simulink model "CalculateMaximumFluxLimit"  (R2026a)
settings: Solver=FixedStepDiscrete
model workspace (MAT data in the model file):
  Polepairs = Simulink.Parameter
  Polepairs.Value = 4
  Polepairs.Complexity = 'real'
  Polepairs.Dimensions = [1 1]
  Polepairs.DataType = 'auto'
settings Model: DataDictionary=TractionEmotorSoftwareArchInterfaceData.sldd  Creator=dakaihu  LastModifiedBy=dakaihu
settings OptimizationCC: GainParamInheritBuiltInType=on  UseFloatMulNetSlope=on  InlineInvariantSignals=on  NoFixptDivByZeroProtection=on  EfficientFloat2IntCast=on  LifeSpan=1
settings HardwareCC: ProdBitPerChar=16.0  ProdBitPerInt=16.0  ProdLargestAtomicInteger=Integer  ProdWordSize=16.0  ProdHWDeviceType=Texas Instruments->C2000
settings RTWCC: SystemTargetFile=ert.tlc  Description=Embedded Coder
settings CodeAppCC: MaxIdLength=60.0  CustomSymbolStrGlobalVar=rt$N$M  CustomSymbolStrType=$N$M  CustomSymbolStrFcn=$N$M$F  CustomSymbolStrMacro=$N$M
settings ERTTargetCC: ERTFilePackagingFormat=CompactWithDataFile  GenerateSampleERTMain=on  IncludeMdlTerminateFcn=off  CombineSignalStateStructs=on  SuppressErrorStatus=on  SupportAbsoluteTime=off  SupportComplex=off

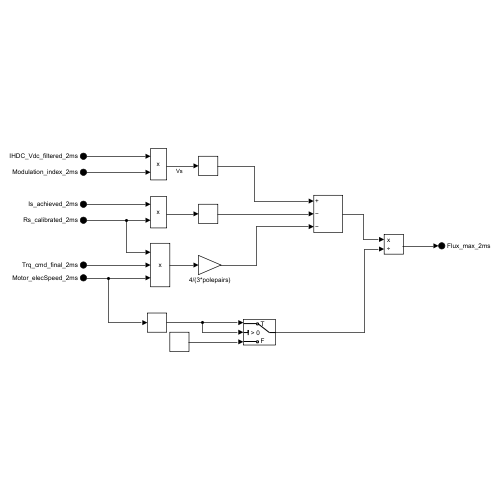
[thumbnail: Simulink's stored preview of the top-level diagram]
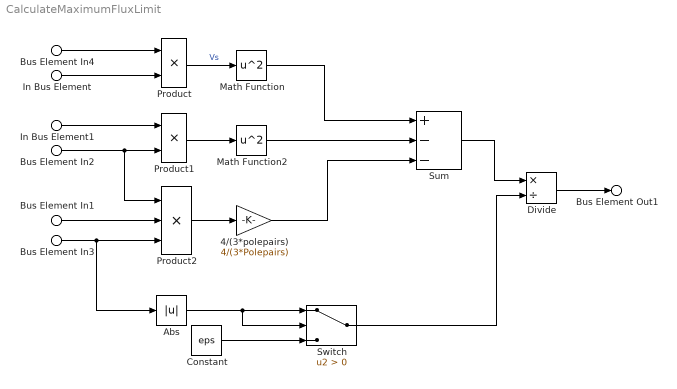
== system CalculateMaximumFluxLimit ==
  Bus Element In2 : Inport  PortName=Rs_calibrated_2ms
  Bus Element In1 : Inport  Port=2  PortName=Trq_cmd_final_2ms
  Bus Element In3 : Inport  Port=3  PortName=Motor_elecSpeed_2ms
  Bus Element In4 : Inport  Port=4  PortName=IHDC_Vdc_filtered_2ms
  In Bus Element : Inport  Port=5  PortName=Modulation_index_2ms
  In Bus Element1 : Inport  Port=6  PortName=Is_achieved_2ms
  4/(3*polepairs) : Gain  Gain=4/(3*Polepairs)
  Abs : Abs  SaturateOnIntegerOverflow=off
  Constant : Constant  Value=eps
  Divide : Product  Inputs=*/
  Math Function : Math  Operator=square
  Math Function2 : Math  Operator=square
  Product : Product
  Product1 : Product
  Product2 : Product  Inputs=3
  Sum : Sum  Inputs=+--
  Switch : Switch  Criteria=u2 > Threshold  SaturateOnIntegerOverflow=off  InputSameDT=off
  Bus Element Out1 : Outport  PortName=Flux_max_2ms
  wires:
  Bus Element In4/1 -> Product/1
  In Bus Element/1 -> Product/2
  Product/1 -> Math Function/1  "Vs"
  In Bus Element1/1 -> Product1/1
  Bus Element In2/1 -> Product2/1, Product1/2
  Product1/1 -> Math Function2/1
  Math Function/1 -> Sum/1
  Math Function2/1 -> Sum/2
  Product2/1 -> 4/(3*polepairs)/1
  4/(3*polepairs)/1 -> Sum/3
  Bus Element In1/1 -> Product2/2
  Sum/1 -> Divide/1
  Divide/1 -> Bus Element Out1/1
  Bus Element In3/1 -> Abs/1, Product2/3
  Switch/1 -> Divide/2
  Constant/1 -> Switch/3
  Abs/1 -> Switch/2, Switch/1
